simulink model "fixedpoint_filter"  (Simulink 7.8)
settings: Solver=ode3  StartTime=0.0  StopTime=1  RelTol=1e-3
values from neighbouring files (symbols this model uses):
  alpha = -7    [reconstruction_filter_setup.m]
  delay_shift2 = -k_preint    (= 0)    [one_bit_control.m]
  fixpt_adder_in_bitwidth = w    (= 24)    [one_bit_control.m]    (also in reconstruction_filter_setup.m)
  fixpt_adder_in_position = d    (= 16)    [one_bit_control.m]    (also in reconstruction_filter_setup.m)
  fixpt_adder_out_bitwidth = w    (= 24)    [one_bit_control.m]    (also in reconstruction_filter_setup.m)
  fixpt_adder_out_position = d    (= 16)    [one_bit_control.m]    (also in reconstruction_filter_setup.m)
  threealpha = 3*alpha    (= -21)    [reconstruction_filter_setup.m]
  ts = 1/Fs    [one_bit_control.m]
libraries: simulink x1
settings Model: Creator=agdibble  LastModifiedBy=agdibble

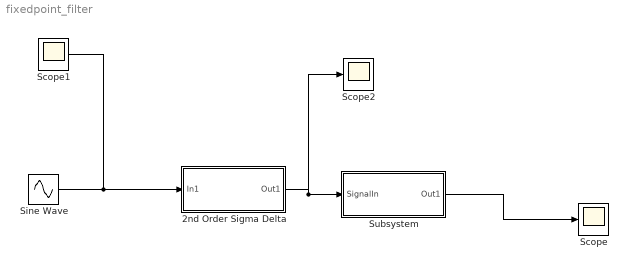
== system fixedpoint_filter ==
  2nd Order Sigma Delta : Subsystem
  Scope : Scope
      settings: YMin=-1.75e-05  YMax=0
  Scope1 : Scope
      settings: YMin=-0.03  YMax=0.03
  Scope2 : Scope
      settings: SaveName=ScopeData2
  Sine Wave : Sin  Amplitude=.03  Frequency=2*pi*10  SampleTime=0
  Subsystem : Subsystem
  wires:
  Sine Wave/1 -> 2nd Order Sigma Delta/1(In1), Scope1/1
  2nd Order Sigma Delta/1(Out1) -> Subsystem/1(SignalIn), Scope2/1
  Subsystem/1(Out1) -> Scope/1

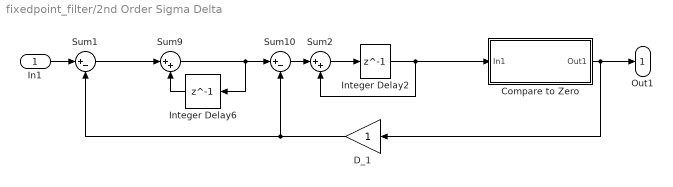
== system fixedpoint_filter/2nd Order Sigma Delta ==
  In1 : Inport
  Compare to Zero : Subsystem
  D_1 : Gain  SampleTime=ts
  Integer Delay2 : Delay  DelayLength=1  InputProcessing=Inherited
  Integer Delay6 : Delay  DelayLength=1  InputProcessing=Inherited
  Sum1 : Sum  Inputs=|+-  SampleTime=ts
  Sum10 : Sum  Inputs=|+-
  Sum2 : Sum  Inputs=|++
  Sum9 : Sum  Inputs=|++  SampleTime=ts
  Out1 : Outport
  wires:
  Sum1/1 -> Sum9/1
  In1/1 -> Sum1/1
  Compare to Zero/1(Out1) -> D_1/1, Out1/1
  Sum2/1 -> Integer Delay2/1
  Integer Delay2/1 -> Sum2/2, Compare to Zero/1(In1)
  Sum9/1 -> Integer Delay6/1, Sum10/1
  Integer Delay6/1 -> Sum9/2
  Sum10/1 -> Sum2/1
  D_1/1 -> Sum1/2, Sum10/2

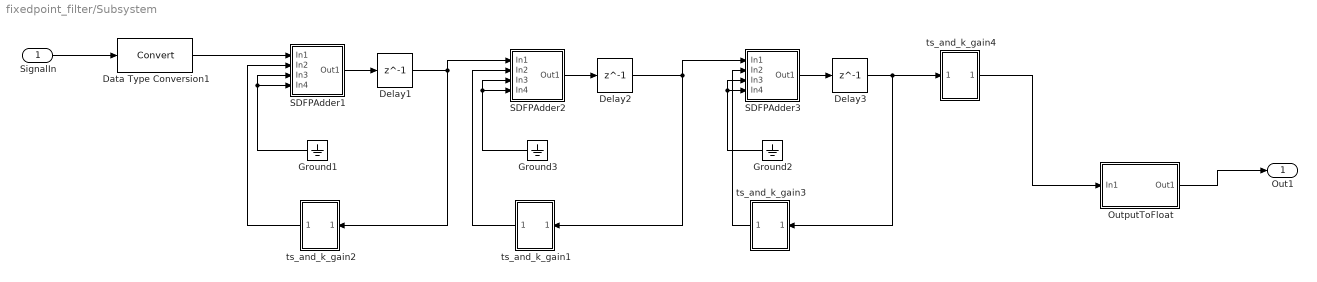
== system fixedpoint_filter/Subsystem ==
  SignalIn : Inport
  Data Type Conversion1 : DataTypeConversion
  Delay1 : Delay  DelayLength=1  InputProcessing=Inherited
  Delay2 : Delay  DelayLength=1  InputProcessing=Inherited
  Delay3 : Delay  DelayLength=1  InputProcessing=Inherited
  Ground1 : Ground
  Ground2 : Ground
  Ground3 : Ground
  OutputToFloat : Subsystem  mask{bitwidth=fixpt_adder_out_bitwidth, fp_position=fixpt_adder_out_position}
      mask prompts: bitwidth "Input Bitwidth"; fp_position "Input Point Position"
      mask Display: disp('Fixed -> Float');
  SDFPAdder1 : Subsystem  mask{in_bitwidth=fixpt_adder_in_bitwidth, in_fp_position=fixpt_adder_in_position, out_bitwidth=fixpt_adder_out_bitwidth, out_fp_position=fixpt_adder_out_position, in1_shift=0, in2_shift=0, in3_shift=0, in4_shift=0}
      mask prompts: in_bitwidth "Input Bitwidth"; in_fp_position "Input Point Position"; out_bitwidth "Output Bitwidth"; out_fp_position "Output Point Position"; in1_shift "Input1 Pre-Shift"; in2_shift "Input2 Pre-Shift"; in3_shift "Input3 Pre-Shift"; in4_shift "Input4 Pre-Shift"
      mask Display: disp(['+\nSDFP'])
  SDFPAdder2 : Subsystem  mask{in_bitwidth=fixpt_adder_in_bitwidth, in_fp_position=fixpt_adder_in_position, out_bitwidth=fixpt_adder_out_bitwidth, out_fp_position=fixpt_adder_out_position, in1_shift=0, in2_shift=0, in3_shift=0, in4_shift=delay_shift2}
      mask prompts: in_bitwidth "Input Bitwidth"; in_fp_position "Input Point Position"; out_bitwidth "Output Bitwidth"; out_fp_position "Output Point Position"; in1_shift "Input1 Pre-Shift"; in2_shift "Input2 Pre-Shift"; in3_shift "Input3 Pre-Shift"; in4_shift "Input4 Pre-Shift"
      mask Display: disp(['+\nSDFP'])
  SDFPAdder3 : Subsystem  mask{in_bitwidth=fixpt_adder_in_bitwidth, in_fp_position=fixpt_adder_in_position, out_bitwidth=fixpt_adder_out_bitwidth, out_fp_position=fixpt_adder_out_position, in1_shift=0, in2_shift=0, in3_shift=0, in4_shift=delay_shift2}
      mask prompts: in_bitwidth "Input Bitwidth"; in_fp_position "Input Point Position"; out_bitwidth "Output Bitwidth"; out_fp_position "Output Point Position"; in1_shift "Input1 Pre-Shift"; in2_shift "Input2 Pre-Shift"; in3_shift "Input3 Pre-Shift"; in4_shift "Input4 Pre-Shift"
      mask Display: disp(['+\nSDFP'])
  ts_and_k_gain1 : Subsystem  mask{shift_amount=alpha}
      mask init:
      | if(shift_amount > 0)
      |     dispval=sprintf('<< %d',shift_amount);
      | else
      |     dispval=sprintf('>> %d',-shift_amount);
      | end
      mask Display: disp(dispval);
  ts_and_k_gain2 : Subsystem  mask{shift_amount=alpha}
      mask init:
      | if(shift_amount > 0)
      |     dispval=sprintf('<< %d',shift_amount);
      | else
      |     dispval=sprintf('>> %d',-shift_amount);
      | end
      mask Display: disp(dispval);
  ts_and_k_gain3 : Subsystem  mask{shift_amount=alpha}
      mask init:
      | if(shift_amount > 0)
      |     dispval=sprintf('<< %d',shift_amount);
      | else
      |     dispval=sprintf('>> %d',-shift_amount);
      | end
      mask Display: disp(dispval);
  ts_and_k_gain4 : Subsystem  mask{shift_amount=threealpha}
      mask init:
      | if(shift_amount > 0)
      |     dispval=sprintf('<< %d',shift_amount);
      | else
      |     dispval=sprintf('>> %d',-shift_amount);
      | end
      mask Display: disp(dispval);
  Out1 : Outport
  wires:
  Ground1/1 -> SDFPAdder1/4(In4), SDFPAdder1/3(In3)
  Ground3/1 -> SDFPAdder2/3(In3), SDFPAdder2/4(In4)
  Ground2/1 -> SDFPAdder3/4(In4), SDFPAdder3/3(In3)
  SDFPAdder2/1(Out1) -> Delay2/1
  SDFPAdder1/1(Out1) -> Delay1/1
  SDFPAdder3/1(Out1) -> Delay3/1
  Delay2/1 -> SDFPAdder3/1(In1), ts_and_k_gain1/1(In1)
  Delay1/1 -> SDFPAdder2/1(In1), ts_and_k_gain2/1(In1)
  ts_and_k_gain3/1(Out1) -> SDFPAdder3/2(In2)
  ts_and_k_gain1/1(Out1) -> SDFPAdder2/2(In2)
  ts_and_k_gain2/1(Out1) -> SDFPAdder1/2(In2)
  Delay3/1 -> ts_and_k_gain3/1(In1), ts_and_k_gain4/1(In1)
  SignalIn/1 -> Data Type Conversion1/1
  Data Type Conversion1/1 -> SDFPAdder1/1(In1)
  OutputToFloat/1(Out1) -> Out1/1
  ts_and_k_gain4/1(Out1) -> OutputToFloat/1(In1)

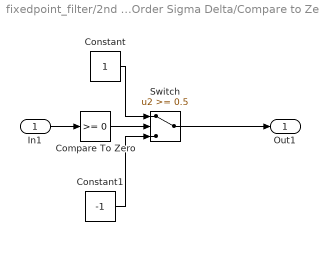
== system fixedpoint_filter/2nd Order Sigma Delta/Compare to Zero ==
  In1 : Inport
  Compare To Zero : simulink/Logic and Bit Operations/Compare To Zero  relop=>=  OutDataTypeStr=uint8
  Constant : Constant
  Constant1 : Constant  Value=-1
  Switch : Switch  Threshold=0.5
  Out1 : Outport
  wires:
  Constant1/1 -> Switch/3
  Constant/1 -> Switch/1
  Compare To Zero/1 -> Switch/2
  In1/1 -> Compare To Zero/1
  Switch/1 -> Out1/1

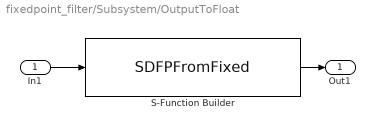
== system fixedpoint_filter/Subsystem/OutputToFloat ==
  In1 : Inport
  S-Function Builder : S-Function  InitFcn=try, set_param(gcb,'FunctionName','SDFPFromFixed'), end  FunctionName=SDFPFromFixed  Parameters=uint32(bitwidth),uint32(fp_position)  SFunctionModules=SDFPFromFixed_wrapper fpconv  WizardData=DataTag0  EnableBusSupport=off  mask(S-Function Builder){}
      mask help: The S-Function Builder block creates a wrapper C-MEX S-function from your supplied C code with multiple input ports, output ports, and a variable number of scalar, vector, or matrix parameters. The input and output ports can propagate Simulink built-in data types, fixed-point datatypes, complex, frame, 1-D, and 2-D signals. This block also supports discrete and continuous states of type real. You can optionally have the block generate a TLC file to be used with Real-Time Workshop for code generation.
      mask init:
      | val = [[.9  0.75 0.75 1 1 .9 .9 1]',[1 1 0.75 0.75 .9 .9 1 .9]'];try , sys = get_param(gcb,'SfunBuilderFcnName');if isempty(sys), sys = get_param(gcb,'FunctionName'); end,catch, sys = get_param(gcb,'FunctionName'); end
      settings: CopyFcn=set_param(gcbh,'LinkStatus','none')  PreSaveFcn=try, set_param(gcb,'FunctionName','SDFPFromFixed'), end  OpenFcn=sfunctionwizard(gcbh)
      mask Display: plot(val(:,1),val(:,2)),disp(sys), port_label('input',1,'fixed_in'), port_label('output',1,'float_out')
  Out1 : Outport
  wires:
  S-Function Builder/1 -> Out1/1
  In1/1 -> S-Function Builder/1

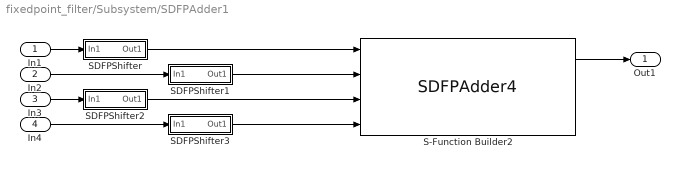
== system fixedpoint_filter/Subsystem/SDFPAdder1 ==
  In1 : Inport
  In2 : Inport  Port=2
  In3 : Inport  Port=3
  In4 : Inport  Port=4
  S-Function Builder2 : S-Function  InitFcn=try, set_param(gcb,'FunctionName','SDFPAdder4'), end  FunctionName=SDFPAdder4  Parameters=uint32(in_bitwidth),uint32(in_fp_position),uint32(out_bitwidth),uint32(out_fp_position)  SFunctionModules=SDFPAdder4_wrapper  WizardData=DataTag1  EnableBusSupport=off  mask(S-Function Builder){}
      mask help: The S-Function Builder block creates a wrapper C-MEX S-function from your supplied C code with multiple input ports, output ports, and a variable number of scalar, vector, or matrix parameters. The input and output ports can propagate Simulink built-in data types, fixed-point datatypes, complex, frame, 1-D, and 2-D signals. This block also supports discrete and continuous states of type real. You can optionally have the block generate a TLC file to be used with Real-Time Workshop for code generation.
      mask init: same as fixedpoint_filter/Subsystem/OutputToFloat/S-Function Builder
      settings: CopyFcn=set_param(gcbh,'LinkStatus','none')  PreSaveFcn=try, set_param(gcb,'FunctionName','SDFPAdder4'), end  OpenFcn=sfunctionwizard(gcbh)
      mask Display: plot(val(:,1),val(:,2)),disp(sys), port_label('input',1,'in0'), port_label('input',2,'in1'), port_label('input',3,'in2'), port_label('input',4,'in3'), port_label('output',1,'adder_out'), port_label('output',2,'DBG_in01'), port_label('output',3,'DBG_in012')
  SDFPShifter : Subsystem  mask{shift_amount=in1_shift}
      mask init:
      | if(shift_amount > 0)
      |     dispval=sprintf('<< %d',shift_amount);
      | else
      |     dispval=sprintf('>> %d',-shift_amount);
      | end
      mask Display: disp(dispval);
  SDFPShifter1 : Subsystem  mask{shift_amount=in2_shift}
      mask init:
      | if(shift_amount > 0)
      |     dispval=sprintf('<< %d',shift_amount);
      | else
      |     dispval=sprintf('>> %d',-shift_amount);
      | end
      mask Display: disp(dispval);
  SDFPShifter2 : Subsystem  mask{shift_amount=in3_shift}
      mask init:
      | if(shift_amount > 0)
      |     dispval=sprintf('<< %d',shift_amount);
      | else
      |     dispval=sprintf('>> %d',-shift_amount);
      | end
      mask Display: disp(dispval);
  SDFPShifter3 : Subsystem  mask{shift_amount=in4_shift}
      mask init:
      | if(shift_amount > 0)
      |     dispval=sprintf('<< %d',shift_amount);
      | else
      |     dispval=sprintf('>> %d',-shift_amount);
      | end
      mask Display: disp(dispval);
  Out1 : Outport
  wires:
  SDFPShifter3/1(Out1) -> S-Function Builder2/4
  SDFPShifter2/1(Out1) -> S-Function Builder2/3
  SDFPShifter1/1(Out1) -> S-Function Builder2/2
  SDFPShifter/1(Out1) -> S-Function Builder2/1
  S-Function Builder2/1 -> Out1/1
  In4/1 -> SDFPShifter3/1(In1)
  In3/1 -> SDFPShifter2/1(In1)
  In2/1 -> SDFPShifter1/1(In1)
  In1/1 -> SDFPShifter/1(In1)

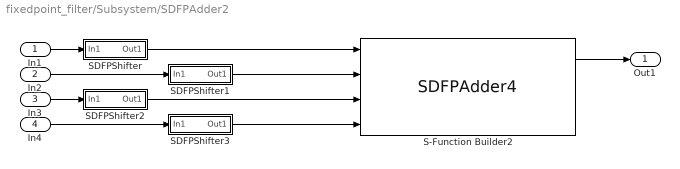
== system fixedpoint_filter/Subsystem/SDFPAdder2 ==
  In1 : Inport
  In2 : Inport  Port=2
  In3 : Inport  Port=3
  In4 : Inport  Port=4
  S-Function Builder2 : S-Function  InitFcn=try, set_param(gcb,'FunctionName','SDFPAdder4'), end  FunctionName=SDFPAdder4  Parameters=uint32(in_bitwidth),uint32(in_fp_position),uint32(out_bitwidth),uint32(out_fp_position)  SFunctionModules=SDFPAdder4_wrapper  WizardData=DataTag6  EnableBusSupport=off  mask(S-Function Builder){}
      mask help: The S-Function Builder block creates a wrapper C-MEX S-function from your supplied C code with multiple input ports, output ports, and a variable number of scalar, vector, or matrix parameters. The input and output ports can propagate Simulink built-in data types, fixed-point datatypes, complex, frame, 1-D, and 2-D signals. This block also supports discrete and continuous states of type real. You can optionally have the block generate a TLC file to be used with Real-Time Workshop for code generation.
      mask init: same as fixedpoint_filter/Subsystem/OutputToFloat/S-Function Builder
      settings: CopyFcn=set_param(gcbh,'LinkStatus','none')  PreSaveFcn=try, set_param(gcb,'FunctionName','SDFPAdder4'), end  OpenFcn=sfunctionwizard(gcbh)
      mask Display: plot(val(:,1),val(:,2)),disp(sys)port_label('input',1,'in0')port_label('input',2,'in1')port_label('input',3,'in2')port_label('input',4,'in3')port_label('output',1,'adder_out')port_label('output',2,'DBG_in01')port_label('output',3,'DBG_in012')
  SDFPShifter : Subsystem  mask{shift_amount=in1_shift}
      mask init:
      | if(shift_amount > 0)
      |     dispval=sprintf('<< %d',shift_amount);
      | else
      |     dispval=sprintf('>> %d',-shift_amount);
      | end
      mask Display: disp(dispval);
  SDFPShifter1 : Subsystem  mask{shift_amount=in2_shift}
      mask init:
      | if(shift_amount > 0)
      |     dispval=sprintf('<< %d',shift_amount);
      | else
      |     dispval=sprintf('>> %d',-shift_amount);
      | end
      mask Display: disp(dispval);
  SDFPShifter2 : Subsystem  mask{shift_amount=in3_shift}
      mask init:
      | if(shift_amount > 0)
      |     dispval=sprintf('<< %d',shift_amount);
      | else
      |     dispval=sprintf('>> %d',-shift_amount);
      | end
      mask Display: disp(dispval);
  SDFPShifter3 : Subsystem  mask{shift_amount=in4_shift}
      mask init:
      | if(shift_amount > 0)
      |     dispval=sprintf('<< %d',shift_amount);
      | else
      |     dispval=sprintf('>> %d',-shift_amount);
      | end
      mask Display: disp(dispval);
  Out1 : Outport
  wires:
  SDFPShifter3/1(Out1) -> S-Function Builder2/4
  SDFPShifter2/1(Out1) -> S-Function Builder2/3
  SDFPShifter1/1(Out1) -> S-Function Builder2/2
  SDFPShifter/1(Out1) -> S-Function Builder2/1
  S-Function Builder2/1 -> Out1/1
  In4/1 -> SDFPShifter3/1(In1)
  In3/1 -> SDFPShifter2/1(In1)
  In2/1 -> SDFPShifter1/1(In1)
  In1/1 -> SDFPShifter/1(In1)

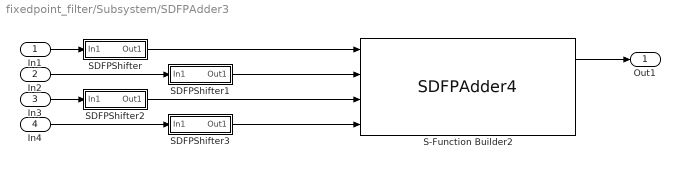
== system fixedpoint_filter/Subsystem/SDFPAdder3 ==
  In1 : Inport
  In2 : Inport  Port=2
  In3 : Inport  Port=3
  In4 : Inport  Port=4
  S-Function Builder2 : S-Function  InitFcn=try, set_param(gcb,'FunctionName','SDFPAdder4'), end  FunctionName=SDFPAdder4  Parameters=uint32(in_bitwidth),uint32(in_fp_position),uint32(out_bitwidth),uint32(out_fp_position)  SFunctionModules=SDFPAdder4_wrapper  WizardData=DataTag11  EnableBusSupport=off  mask(S-Function Builder){}
      mask help: The S-Function Builder block creates a wrapper C-MEX S-function from your supplied C code with multiple input ports, output ports, and a variable number of scalar, vector, or matrix parameters. The input and output ports can propagate Simulink built-in data types, fixed-point datatypes, complex, frame, 1-D, and 2-D signals. This block also supports discrete and continuous states of type real. You can optionally have the block generate a TLC file to be used with Real-Time Workshop for code generation.
      mask init: same as fixedpoint_filter/Subsystem/OutputToFloat/S-Function Builder
      settings: CopyFcn=set_param(gcbh,'LinkStatus','none')  PreSaveFcn=try, set_param(gcb,'FunctionName','SDFPAdder4'), end  OpenFcn=sfunctionwizard(gcbh)
      mask Display: plot(val(:,1),val(:,2)),disp(sys)port_label('input',1,'in0')port_label('input',2,'in1')port_label('input',3,'in2')port_label('input',4,'in3')port_label('output',1,'adder_out')port_label('output',2,'DBG_in01')port_label('output',3,'DBG_in012')
  SDFPShifter : Subsystem  mask{shift_amount=in1_shift}
      mask init:
      | if(shift_amount > 0)
      |     dispval=sprintf('<< %d',shift_amount);
      | else
      |     dispval=sprintf('>> %d',-shift_amount);
      | end
      mask Display: disp(dispval);
  SDFPShifter1 : Subsystem  mask{shift_amount=in2_shift}
      mask init:
      | if(shift_amount > 0)
      |     dispval=sprintf('<< %d',shift_amount);
      | else
      |     dispval=sprintf('>> %d',-shift_amount);
      | end
      mask Display: disp(dispval);
  SDFPShifter2 : Subsystem  mask{shift_amount=in3_shift}
      mask init:
      | if(shift_amount > 0)
      |     dispval=sprintf('<< %d',shift_amount);
      | else
      |     dispval=sprintf('>> %d',-shift_amount);
      | end
      mask Display: disp(dispval);
  SDFPShifter3 : Subsystem  mask{shift_amount=in4_shift}
      mask init:
      | if(shift_amount > 0)
      |     dispval=sprintf('<< %d',shift_amount);
      | else
      |     dispval=sprintf('>> %d',-shift_amount);
      | end
      mask Display: disp(dispval);
  Out1 : Outport
  wires:
  SDFPShifter3/1(Out1) -> S-Function Builder2/4
  SDFPShifter2/1(Out1) -> S-Function Builder2/3
  SDFPShifter1/1(Out1) -> S-Function Builder2/2
  SDFPShifter/1(Out1) -> S-Function Builder2/1
  S-Function Builder2/1 -> Out1/1
  In4/1 -> SDFPShifter3/1(In1)
  In3/1 -> SDFPShifter2/1(In1)
  In2/1 -> SDFPShifter1/1(In1)
  In1/1 -> SDFPShifter/1(In1)

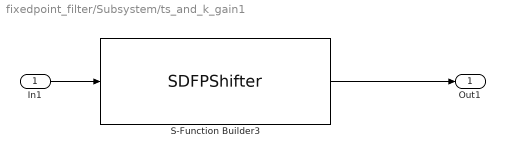
== system fixedpoint_filter/Subsystem/ts_and_k_gain1 ==
  In1 : Inport
  S-Function Builder3 : S-Function  InitFcn=try, set_param(gcb,'FunctionName','SDFPShifter'), end  FunctionName=SDFPShifter  Parameters=int32(shift_amount)  SFunctionModules=SDFPShifter_wrapper  WizardData=DataTag16  EnableBusSupport=off  mask(S-Function Builder){}
      mask help: The S-Function Builder block creates a wrapper C-MEX S-function from your supplied C code with multiple input ports, output ports, and a variable number of scalar, vector, or matrix parameters. The input and output ports can propagate Simulink built-in data types, fixed-point datatypes, complex, frame, 1-D, and 2-D signals. This block also supports discrete and continuous states of type real. You can optionally have the block generate a TLC file to be used with Real-Time Workshop for code generation.
      mask init: same as fixedpoint_filter/Subsystem/OutputToFloat/S-Function Builder
      settings: CopyFcn=set_param(gcbh,'LinkStatus','none')  PreSaveFcn=try, set_param(gcb,'FunctionName','SDFPShifter'), end  OpenFcn=sfunctionwizard(gcbh)
      mask Display: plot(val(:,1),val(:,2)),disp(sys)port_label('input',1,'sg_in')port_label('output',1,'shifter_out')
  Out1 : Outport
  wires:
  S-Function Builder3/1 -> Out1/1
  In1/1 -> S-Function Builder3/1

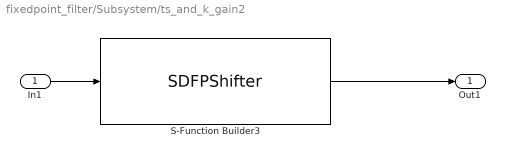
== system fixedpoint_filter/Subsystem/ts_and_k_gain2 ==
  In1 : Inport
  S-Function Builder3 : S-Function  InitFcn=try, set_param(gcb,'FunctionName','SDFPShifter'), end  FunctionName=SDFPShifter  Parameters=int32(shift_amount)  SFunctionModules=SDFPShifter_wrapper  WizardData=DataTag17  EnableBusSupport=off  mask(S-Function Builder){}
      mask help: The S-Function Builder block creates a wrapper C-MEX S-function from your supplied C code with multiple input ports, output ports, and a variable number of scalar, vector, or matrix parameters. The input and output ports can propagate Simulink built-in data types, fixed-point datatypes, complex, frame, 1-D, and 2-D signals. This block also supports discrete and continuous states of type real. You can optionally have the block generate a TLC file to be used with Real-Time Workshop for code generation.
      mask init: same as fixedpoint_filter/Subsystem/OutputToFloat/S-Function Builder
      settings: CopyFcn=set_param(gcbh,'LinkStatus','none')  PreSaveFcn=try, set_param(gcb,'FunctionName','SDFPShifter'), end  OpenFcn=sfunctionwizard(gcbh)
      mask Display: plot(val(:,1),val(:,2)),disp(sys)port_label('input',1,'sg_in')port_label('output',1,'shifter_out')
  Out1 : Outport
  wires:
  S-Function Builder3/1 -> Out1/1
  In1/1 -> S-Function Builder3/1

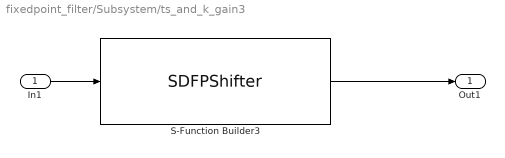
== system fixedpoint_filter/Subsystem/ts_and_k_gain3 ==
  In1 : Inport
  S-Function Builder3 : S-Function  InitFcn=try, set_param(gcb,'FunctionName','SDFPShifter'), end  FunctionName=SDFPShifter  Parameters=int32(shift_amount)  SFunctionModules=SDFPShifter_wrapper  WizardData=DataTag18  EnableBusSupport=off  mask(S-Function Builder){}
      mask help: The S-Function Builder block creates a wrapper C-MEX S-function from your supplied C code with multiple input ports, output ports, and a variable number of scalar, vector, or matrix parameters. The input and output ports can propagate Simulink built-in data types, fixed-point datatypes, complex, frame, 1-D, and 2-D signals. This block also supports discrete and continuous states of type real. You can optionally have the block generate a TLC file to be used with Real-Time Workshop for code generation.
      mask init: same as fixedpoint_filter/Subsystem/OutputToFloat/S-Function Builder
      settings: CopyFcn=set_param(gcbh,'LinkStatus','none')  PreSaveFcn=try, set_param(gcb,'FunctionName','SDFPShifter'), end  OpenFcn=sfunctionwizard(gcbh)
      mask Display: plot(val(:,1),val(:,2)),disp(sys)port_label('input',1,'sg_in')port_label('output',1,'shifter_out')
  Out1 : Outport
  wires:
  S-Function Builder3/1 -> Out1/1
  In1/1 -> S-Function Builder3/1

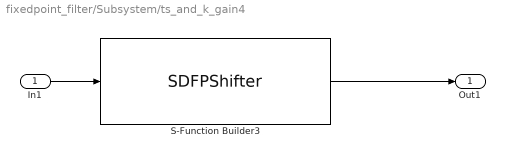
== system fixedpoint_filter/Subsystem/ts_and_k_gain4 ==
  In1 : Inport
  S-Function Builder3 : S-Function  InitFcn=try, set_param(gcb,'FunctionName','SDFPShifter'), end  FunctionName=SDFPShifter  Parameters=int32(shift_amount)  SFunctionModules=SDFPShifter_wrapper  WizardData=DataTag19  EnableBusSupport=off  mask(S-Function Builder){}
      mask help: The S-Function Builder block creates a wrapper C-MEX S-function from your supplied C code with multiple input ports, output ports, and a variable number of scalar, vector, or matrix parameters. The input and output ports can propagate Simulink built-in data types, fixed-point datatypes, complex, frame, 1-D, and 2-D signals. This block also supports discrete and continuous states of type real. You can optionally have the block generate a TLC file to be used with Real-Time Workshop for code generation.
      mask init: same as fixedpoint_filter/Subsystem/OutputToFloat/S-Function Builder
      settings: CopyFcn=set_param(gcbh,'LinkStatus','none')  PreSaveFcn=try, set_param(gcb,'FunctionName','SDFPShifter'), end  OpenFcn=sfunctionwizard(gcbh)
      mask Display: plot(val(:,1),val(:,2)),disp(sys)port_label('input',1,'sg_in')port_label('output',1,'shifter_out')
  Out1 : Outport
  wires:
  S-Function Builder3/1 -> Out1/1
  In1/1 -> S-Function Builder3/1

== system fixedpoint_filter/Subsystem/SDFPAdder1/SDFPShifter ==
  In1 : Inport
  S-Function Builder3 : S-Function  InitFcn=try, set_param(gcb,'FunctionName','SDFPShifter'), end  FunctionName=SDFPShifter  Parameters=int32(shift_amount)  SFunctionModules=SDFPShifter_wrapper  WizardData=DataTag2  EnableBusSupport=off  mask(S-Function Builder){}
      mask help: The S-Function Builder block creates a wrapper C-MEX S-function from your supplied C code with multiple input ports, output ports, and a variable number of scalar, vector, or matrix parameters. The input and output ports can propagate Simulink built-in data types, fixed-point datatypes, complex, frame, 1-D, and 2-D signals. This block also supports discrete and continuous states of type real. You can optionally have the block generate a TLC file to be used with Real-Time Workshop for code generation.
      mask init: same as fixedpoint_filter/Subsystem/OutputToFloat/S-Function Builder
      settings: CopyFcn=set_param(gcbh,'LinkStatus','none')  PreSaveFcn=try, set_param(gcb,'FunctionName','SDFPShifter'), end  OpenFcn=sfunctionwizard(gcbh)
      mask Display: plot(val(:,1),val(:,2)),disp(sys), port_label('input',1,'sg_in'), port_label('output',1,'shifter_out')
  Out1 : Outport
  wires:
  S-Function Builder3/1 -> Out1/1
  In1/1 -> S-Function Builder3/1

== system fixedpoint_filter/Subsystem/SDFPAdder1/SDFPShifter1 ==
  In1 : Inport
  S-Function Builder3 : S-Function  InitFcn=try, set_param(gcb,'FunctionName','SDFPShifter'), end  FunctionName=SDFPShifter  Parameters=int32(shift_amount)  SFunctionModules=SDFPShifter_wrapper  WizardData=DataTag3  EnableBusSupport=off  mask(S-Function Builder){}
      mask help: The S-Function Builder block creates a wrapper C-MEX S-function from your supplied C code with multiple input ports, output ports, and a variable number of scalar, vector, or matrix parameters. The input and output ports can propagate Simulink built-in data types, fixed-point datatypes, complex, frame, 1-D, and 2-D signals. This block also supports discrete and continuous states of type real. You can optionally have the block generate a TLC file to be used with Real-Time Workshop for code generation.
      mask init: same as fixedpoint_filter/Subsystem/OutputToFloat/S-Function Builder
      settings: CopyFcn=set_param(gcbh,'LinkStatus','none')  PreSaveFcn=try, set_param(gcb,'FunctionName','SDFPShifter'), end  OpenFcn=sfunctionwizard(gcbh)
      mask Display: plot(val(:,1),val(:,2)),disp(sys)port_label('input',1,'sg_in')port_label('output',1,'shifter_out')
  Out1 : Outport
  wires:
  In1/1 -> S-Function Builder3/1
  S-Function Builder3/1 -> Out1/1

== system fixedpoint_filter/Subsystem/SDFPAdder1/SDFPShifter2 ==
  In1 : Inport
  S-Function Builder3 : S-Function  InitFcn=try, set_param(gcb,'FunctionName','SDFPShifter'), end  FunctionName=SDFPShifter  Parameters=int32(shift_amount)  SFunctionModules=SDFPShifter_wrapper  WizardData=DataTag4  EnableBusSupport=off  mask(S-Function Builder){}
      mask help: The S-Function Builder block creates a wrapper C-MEX S-function from your supplied C code with multiple input ports, output ports, and a variable number of scalar, vector, or matrix parameters. The input and output ports can propagate Simulink built-in data types, fixed-point datatypes, complex, frame, 1-D, and 2-D signals. This block also supports discrete and continuous states of type real. You can optionally have the block generate a TLC file to be used with Real-Time Workshop for code generation.
      mask init: same as fixedpoint_filter/Subsystem/OutputToFloat/S-Function Builder
      settings: CopyFcn=set_param(gcbh,'LinkStatus','none')  PreSaveFcn=try, set_param(gcb,'FunctionName','SDFPShifter'), end  OpenFcn=sfunctionwizard(gcbh)
      mask Display: plot(val(:,1),val(:,2)),disp(sys)port_label('input',1,'sg_in')port_label('output',1,'shifter_out')
  Out1 : Outport
  wires:
  S-Function Builder3/1 -> Out1/1
  In1/1 -> S-Function Builder3/1

== system fixedpoint_filter/Subsystem/SDFPAdder1/SDFPShifter3 ==
  In1 : Inport
  S-Function Builder3 : S-Function  InitFcn=try, set_param(gcb,'FunctionName','SDFPShifter'), end  FunctionName=SDFPShifter  Parameters=int32(shift_amount)  SFunctionModules=SDFPShifter_wrapper  WizardData=DataTag5  EnableBusSupport=off  mask(S-Function Builder){}
      mask help: The S-Function Builder block creates a wrapper C-MEX S-function from your supplied C code with multiple input ports, output ports, and a variable number of scalar, vector, or matrix parameters. The input and output ports can propagate Simulink built-in data types, fixed-point datatypes, complex, frame, 1-D, and 2-D signals. This block also supports discrete and continuous states of type real. You can optionally have the block generate a TLC file to be used with Real-Time Workshop for code generation.
      mask init: same as fixedpoint_filter/Subsystem/OutputToFloat/S-Function Builder
      settings: CopyFcn=set_param(gcbh,'LinkStatus','none')  PreSaveFcn=try, set_param(gcb,'FunctionName','SDFPShifter'), end  OpenFcn=sfunctionwizard(gcbh)
      mask Display: plot(val(:,1),val(:,2)),disp(sys)port_label('input',1,'sg_in')port_label('output',1,'shifter_out')
  Out1 : Outport
  wires:
  In1/1 -> S-Function Builder3/1
  S-Function Builder3/1 -> Out1/1

== system fixedpoint_filter/Subsystem/SDFPAdder2/SDFPShifter ==
  In1 : Inport
  S-Function Builder3 : S-Function  InitFcn=try, set_param(gcb,'FunctionName','SDFPShifter'), end  FunctionName=SDFPShifter  Parameters=int32(shift_amount)  SFunctionModules=SDFPShifter_wrapper  WizardData=DataTag7  EnableBusSupport=off  mask(S-Function Builder){}
      mask help: The S-Function Builder block creates a wrapper C-MEX S-function from your supplied C code with multiple input ports, output ports, and a variable number of scalar, vector, or matrix parameters. The input and output ports can propagate Simulink built-in data types, fixed-point datatypes, complex, frame, 1-D, and 2-D signals. This block also supports discrete and continuous states of type real. You can optionally have the block generate a TLC file to be used with Real-Time Workshop for code generation.
      mask init: same as fixedpoint_filter/Subsystem/OutputToFloat/S-Function Builder
      settings: CopyFcn=set_param(gcbh,'LinkStatus','none')  PreSaveFcn=try, set_param(gcb,'FunctionName','SDFPShifter'), end  OpenFcn=sfunctionwizard(gcbh)
      mask Display: plot(val(:,1),val(:,2)),disp(sys)port_label('input',1,'sg_in')port_label('output',1,'shifter_out')
  Out1 : Outport
  wires:
  S-Function Builder3/1 -> Out1/1
  In1/1 -> S-Function Builder3/1

== system fixedpoint_filter/Subsystem/SDFPAdder2/SDFPShifter1 ==
  In1 : Inport
  S-Function Builder3 : S-Function  InitFcn=try, set_param(gcb,'FunctionName','SDFPShifter'), end  FunctionName=SDFPShifter  Parameters=int32(shift_amount)  SFunctionModules=SDFPShifter_wrapper  WizardData=DataTag8  EnableBusSupport=off  mask(S-Function Builder){}
      mask help: The S-Function Builder block creates a wrapper C-MEX S-function from your supplied C code with multiple input ports, output ports, and a variable number of scalar, vector, or matrix parameters. The input and output ports can propagate Simulink built-in data types, fixed-point datatypes, complex, frame, 1-D, and 2-D signals. This block also supports discrete and continuous states of type real. You can optionally have the block generate a TLC file to be used with Real-Time Workshop for code generation.
      mask init: same as fixedpoint_filter/Subsystem/OutputToFloat/S-Function Builder
      settings: CopyFcn=set_param(gcbh,'LinkStatus','none')  PreSaveFcn=try, set_param(gcb,'FunctionName','SDFPShifter'), end  OpenFcn=sfunctionwizard(gcbh)
      mask Display: plot(val(:,1),val(:,2)),disp(sys)port_label('input',1,'sg_in')port_label('output',1,'shifter_out')
  Out1 : Outport
  wires:
  In1/1 -> S-Function Builder3/1
  S-Function Builder3/1 -> Out1/1

== system fixedpoint_filter/Subsystem/SDFPAdder2/SDFPShifter2 ==
  In1 : Inport
  S-Function Builder3 : S-Function  InitFcn=try, set_param(gcb,'FunctionName','SDFPShifter'), end  FunctionName=SDFPShifter  Parameters=int32(shift_amount)  SFunctionModules=SDFPShifter_wrapper  WizardData=DataTag9  EnableBusSupport=off  mask(S-Function Builder){}
      mask help: The S-Function Builder block creates a wrapper C-MEX S-function from your supplied C code with multiple input ports, output ports, and a variable number of scalar, vector, or matrix parameters. The input and output ports can propagate Simulink built-in data types, fixed-point datatypes, complex, frame, 1-D, and 2-D signals. This block also supports discrete and continuous states of type real. You can optionally have the block generate a TLC file to be used with Real-Time Workshop for code generation.
      mask init: same as fixedpoint_filter/Subsystem/OutputToFloat/S-Function Builder
      settings: CopyFcn=set_param(gcbh,'LinkStatus','none')  PreSaveFcn=try, set_param(gcb,'FunctionName','SDFPShifter'), end  OpenFcn=sfunctionwizard(gcbh)
      mask Display: plot(val(:,1),val(:,2)),disp(sys)port_label('input',1,'sg_in')port_label('output',1,'shifter_out')
  Out1 : Outport
  wires:
  S-Function Builder3/1 -> Out1/1
  In1/1 -> S-Function Builder3/1

== system fixedpoint_filter/Subsystem/SDFPAdder2/SDFPShifter3 ==
  In1 : Inport
  S-Function Builder3 : S-Function  InitFcn=try, set_param(gcb,'FunctionName','SDFPShifter'), end  FunctionName=SDFPShifter  Parameters=int32(shift_amount)  SFunctionModules=SDFPShifter_wrapper  WizardData=DataTag10  EnableBusSupport=off  mask(S-Function Builder){}
      mask help: The S-Function Builder block creates a wrapper C-MEX S-function from your supplied C code with multiple input ports, output ports, and a variable number of scalar, vector, or matrix parameters. The input and output ports can propagate Simulink built-in data types, fixed-point datatypes, complex, frame, 1-D, and 2-D signals. This block also supports discrete and continuous states of type real. You can optionally have the block generate a TLC file to be used with Real-Time Workshop for code generation.
      mask init: same as fixedpoint_filter/Subsystem/OutputToFloat/S-Function Builder
      settings: CopyFcn=set_param(gcbh,'LinkStatus','none')  PreSaveFcn=try, set_param(gcb,'FunctionName','SDFPShifter'), end  OpenFcn=sfunctionwizard(gcbh)
      mask Display: plot(val(:,1),val(:,2)),disp(sys)port_label('input',1,'sg_in')port_label('output',1,'shifter_out')
  Out1 : Outport
  wires:
  In1/1 -> S-Function Builder3/1
  S-Function Builder3/1 -> Out1/1

== system fixedpoint_filter/Subsystem/SDFPAdder3/SDFPShifter ==
  In1 : Inport
  S-Function Builder3 : S-Function  InitFcn=try, set_param(gcb,'FunctionName','SDFPShifter'), end  FunctionName=SDFPShifter  Parameters=int32(shift_amount)  SFunctionModules=SDFPShifter_wrapper  WizardData=DataTag12  EnableBusSupport=off  mask(S-Function Builder){}
      mask help: The S-Function Builder block creates a wrapper C-MEX S-function from your supplied C code with multiple input ports, output ports, and a variable number of scalar, vector, or matrix parameters. The input and output ports can propagate Simulink built-in data types, fixed-point datatypes, complex, frame, 1-D, and 2-D signals. This block also supports discrete and continuous states of type real. You can optionally have the block generate a TLC file to be used with Real-Time Workshop for code generation.
      mask init: same as fixedpoint_filter/Subsystem/OutputToFloat/S-Function Builder
      settings: CopyFcn=set_param(gcbh,'LinkStatus','none')  PreSaveFcn=try, set_param(gcb,'FunctionName','SDFPShifter'), end  OpenFcn=sfunctionwizard(gcbh)
      mask Display: plot(val(:,1),val(:,2)),disp(sys)port_label('input',1,'sg_in')port_label('output',1,'shifter_out')
  Out1 : Outport
  wires:
  S-Function Builder3/1 -> Out1/1
  In1/1 -> S-Function Builder3/1

== system fixedpoint_filter/Subsystem/SDFPAdder3/SDFPShifter1 ==
  In1 : Inport
  S-Function Builder3 : S-Function  InitFcn=try, set_param(gcb,'FunctionName','SDFPShifter'), end  FunctionName=SDFPShifter  Parameters=int32(shift_amount)  SFunctionModules=SDFPShifter_wrapper  WizardData=DataTag13  EnableBusSupport=off  mask(S-Function Builder){}
      mask help: The S-Function Builder block creates a wrapper C-MEX S-function from your supplied C code with multiple input ports, output ports, and a variable number of scalar, vector, or matrix parameters. The input and output ports can propagate Simulink built-in data types, fixed-point datatypes, complex, frame, 1-D, and 2-D signals. This block also supports discrete and continuous states of type real. You can optionally have the block generate a TLC file to be used with Real-Time Workshop for code generation.
      mask init: same as fixedpoint_filter/Subsystem/OutputToFloat/S-Function Builder
      settings: CopyFcn=set_param(gcbh,'LinkStatus','none')  PreSaveFcn=try, set_param(gcb,'FunctionName','SDFPShifter'), end  OpenFcn=sfunctionwizard(gcbh)
      mask Display: plot(val(:,1),val(:,2)),disp(sys)port_label('input',1,'sg_in')port_label('output',1,'shifter_out')
  Out1 : Outport
  wires:
  In1/1 -> S-Function Builder3/1
  S-Function Builder3/1 -> Out1/1

== system fixedpoint_filter/Subsystem/SDFPAdder3/SDFPShifter2 ==
  In1 : Inport
  S-Function Builder3 : S-Function  InitFcn=try, set_param(gcb,'FunctionName','SDFPShifter'), end  FunctionName=SDFPShifter  Parameters=int32(shift_amount)  SFunctionModules=SDFPShifter_wrapper  WizardData=DataTag14  EnableBusSupport=off  mask(S-Function Builder){}
      mask help: The S-Function Builder block creates a wrapper C-MEX S-function from your supplied C code with multiple input ports, output ports, and a variable number of scalar, vector, or matrix parameters. The input and output ports can propagate Simulink built-in data types, fixed-point datatypes, complex, frame, 1-D, and 2-D signals. This block also supports discrete and continuous states of type real. You can optionally have the block generate a TLC file to be used with Real-Time Workshop for code generation.
      mask init: same as fixedpoint_filter/Subsystem/OutputToFloat/S-Function Builder
      settings: CopyFcn=set_param(gcbh,'LinkStatus','none')  PreSaveFcn=try, set_param(gcb,'FunctionName','SDFPShifter'), end  OpenFcn=sfunctionwizard(gcbh)
      mask Display: plot(val(:,1),val(:,2)),disp(sys)port_label('input',1,'sg_in')port_label('output',1,'shifter_out')
  Out1 : Outport
  wires:
  S-Function Builder3/1 -> Out1/1
  In1/1 -> S-Function Builder3/1

== system fixedpoint_filter/Subsystem/SDFPAdder3/SDFPShifter3 ==
  In1 : Inport
  S-Function Builder3 : S-Function  InitFcn=try, set_param(gcb,'FunctionName','SDFPShifter'), end  FunctionName=SDFPShifter  Parameters=int32(shift_amount)  SFunctionModules=SDFPShifter_wrapper  WizardData=DataTag15  EnableBusSupport=off  mask(S-Function Builder){}
      mask help: The S-Function Builder block creates a wrapper C-MEX S-function from your supplied C code with multiple input ports, output ports, and a variable number of scalar, vector, or matrix parameters. The input and output ports can propagate Simulink built-in data types, fixed-point datatypes, complex, frame, 1-D, and 2-D signals. This block also supports discrete and continuous states of type real. You can optionally have the block generate a TLC file to be used with Real-Time Workshop for code generation.
      mask init: same as fixedpoint_filter/Subsystem/OutputToFloat/S-Function Builder
      settings: CopyFcn=set_param(gcbh,'LinkStatus','none')  PreSaveFcn=try, set_param(gcb,'FunctionName','SDFPShifter'), end  OpenFcn=sfunctionwizard(gcbh)
      mask Display: plot(val(:,1),val(:,2)),disp(sys)port_label('input',1,'sg_in')port_label('output',1,'shifter_out')
  Out1 : Outport
  wires:
  In1/1 -> S-Function Builder3/1
  S-Function Builder3/1 -> Out1/1
